simulink model "LQR"  (R2024b)
settings: Solver=VariableStepAuto  StartTime=0.0  StopTime=20  RelTol=1e-3
settings Model: Creator=12625  LastModifiedBy=12625

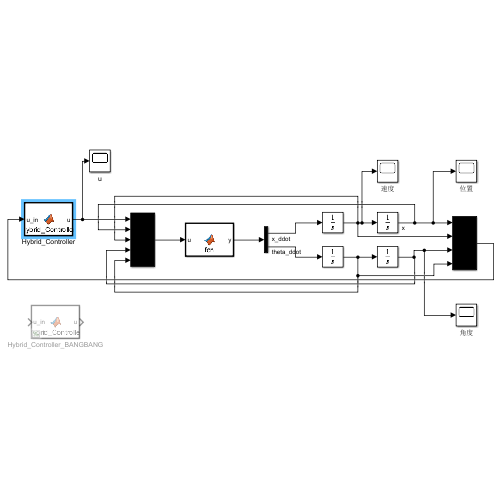
[thumbnail: Simulink's stored preview of the top-level diagram]
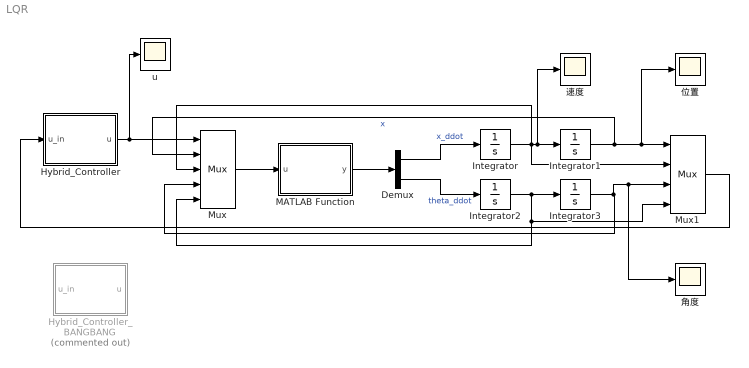
== system LQR ==
  Demux : Demux  Outputs=2
  Hybrid_Controller : MATLAB Function  TreatAsAtomicUnit=on
  Hybrid_Controller_BANGBANG : MATLAB Function  Commented=on  TreatAsAtomicUnit=on
  Integrator : Integrator
  Integrator1 : Integrator
  Integrator2 : Integrator
  Integrator3 : Integrator  InitialCondition=-3.14
  MATLAB Function : MATLAB Function  TreatAsAtomicUnit=on
  Mux : Mux  Inputs=5
  Mux1 : Mux
  u : Scope
  位置 : Scope
  角度 : Scope
  速度 : Scope
  wires:
  Demux/1 -> Integrator/1  "x_ddot"
  Integrator/1 -> Mux1/2, Mux/3, 速度/1, Integrator1/1
  Demux/2 -> Integrator2/1  "theta_ddot"
  Integrator2/1 -> Mux1/4, Mux/5, Integrator3/1
  MATLAB Function/1(y) -> Demux/1
  Integrator1/1 -> 位置/1, Mux1/1, Mux/2  "x"
  Integrator3/1 -> 角度/1, Mux1/3, Mux/4
  Mux1/1 -> Hybrid_Controller/1(u_in)
  Hybrid_Controller/1(u) -> u/1, Mux/1
  Mux/1 -> MATLAB Function/1(u)

== matlab function LQR/MATLAB Function ==
  data: y output; u input
function y = fcn(u)
% 输入 u 包含: [F, x, x_dot, theta, theta_dot]
% 输出 y 包含: [x_ddot, theta_ddot]

% 1. 解包输入
F = u(1);
% x = u(2); % 其实方程里没用到x，只需要速度和角度
x_dot = u(3);
theta = u(4);
theta_dot = u(5);

% 2. 定义参数 (一定要和你的推导一致)
M = 0.5;  % 小车质量
m = 0.2;  % 摆杆质量
l = 0.5;  % 杆长的一半
g = 9.8;
I = 0.005; % 假设均匀杆 I = 1/12*m*(2l)^2 approx

% 3. 写入刚才推导出的公式 (这里用标准形式)
% 这里的公式是为了解出 x_ddot 和 theta_ddot
% 我们可以构建一个矩阵方程 Ax=b 来解，或者直接写解析解
% 为了简单，这里直接写解好的形式 (分母项)

sin_t = sin(theta);
cos_t = cos(theta);
denom = (M+m)*(I+m*l^2) - (m*l*cos_t)^2;

% 分子项
term1 = (I+m*l^2)*F + (I+m*l^2)*m*l*theta_dot^2*sin_t - m*l*cos_t*m*g*sin_t;
term2 = (M+m)*m*g*sin_t - m*l*cos_t*F - m*l*cos_t*m*l*theta_dot^2*sin_t;

x_ddot = term1 / denom;
theta_ddot = term2 / denom;

y = [x_ddot; theta_ddot];

== matlab function LQR/Hybrid_Controller_BANGBANG ==
  data: u output; u_in input
function u = Hybrid_Controller(u_in)
    % 解包输入
    x = u_in(1);
    x_dot = u_in(2);
    theta = u_in(3);     % 原始角度
    theta_dot = u_in(4);
    
    % --- 1. 参数定义 ---
    M = 1.0; m = 0.1; l = 0.5; g = 9.8;
    I_cm = 0.005;
    J = I_cm + m*l^2;
    
    % --- 2. 角度归一化 ---
    theta_norm = mod(theta + pi, 2*pi) - pi;
    
    % --- 3. 能量计算 ---
    E_ref = m * g * l; 
    E_now = 0.5 * J * theta_dot^2 + m * g * l * cos(theta_norm);
    E_err = E_now - E_ref;


    
    % --- 4. 状态机切换逻辑 ---
    if abs(theta_norm) < 0.45
        % === 状态 A: LQR 稳态控制 ===
        K = [-1.0000   ,-3.4655  ,-73.5731  ,-11.5865]; 
        
        state_vec = [x; x_dot; theta_norm; theta_dot];
        u = -K * state_vec;
        
        % LQR 限幅
        u = max(min(u, 20), -20);
        
    else
        % === 状态 B: Swing-Up "慢速安全起摆" ===
        
        % 1. 安全区设置 (保持严格)
        % 只要跑出 0.3米，就开始报警准备救车
        safe_zone_limit = 0.3; 
        
        % 2. 降低推力 (解决 2.5米 的核心)
        % 从 12.0 降到 6.0。
        % 宁可让它多摆 5 秒钟，也不要让车跑太快。
        pump_force = 6.0; 
        
        % 计算推力方向 (Bang-Bang 控制)
        u_swing_direction = -sign(theta_dot * cos(theta_norm));
        u_swing = pump_force * u_swing_direction;
        
        % --- 3. 核心调度 ---
        if abs(x) > safe_zone_limit
            % [红区]：急刹车 (救车模式)
            k_safe_pos = 8.0;  % 强拉力
            k_safe_vel = 5.0;  % 强阻尼
            
            u = - (k_safe_pos * x + k_safe_vel * x_dot);
            
        else
            % [绿区]：带阻尼的起摆 (关键修改!)
            
            % 以前是 u = u_swing; (无阻力)
            % 现在减去速度项 (2.0 * x_dot)。
            % 这就像车轮带点刹车，防止在起摆过程中车速飙升。
            u = u_swing - (2.5 * x_dot); 
        end
        
        % 4. 限幅
        u = max(min(u, 25), -25); 
    end
end

== matlab function LQR/Hybrid_Controller ==
  data: u output; u_in input
function u = Hybrid_Controller(u_in)
    % 解包输入
    x = u_in(1);
    x_dot = u_in(2);
    theta = u_in(3);     
    theta_dot = u_in(4);
    
    % --- 1. 参数定义 (必须与脚本里的黄金参数一致！) ---
    M = 0.5;  % 小车变轻
    m = 0.2;  % 摆杆变重
    l = 0.5;  
    g = 9.8;
    I_cm = 0.005; 
    
    % --- 2. 角度归一化 ---
    theta_norm = mod(theta + pi, 2*pi) - pi;
    
    % --- 3. 能量计算 ---
    J = I_cm + m*l^2;
    E_ref = 0.97*m * g * l; 
    E_now = 0.5 * J * theta_dot^2 + m * g * l * cos(theta_norm);
    
    % --- 4. 状态机切换 ---
    % 只要进入 20度 (0.35 rad) 范围内，就切 LQR
    if abs(theta_norm) < 0.45
        % === 状态 A: LQR 稳态控制 ===
        % 【注意】这里必须用你刚才脚本算出来的新 K 值！
        % 我这里放一个大概的估计值，请用脚本算出的覆盖它
        % 假设 K_new 类似这样 (请务必更新):
        K = [-99.999999999998950,-51.470097958987274,-2.194250822195372e+02,-39.883194125206046]; % <--- 记得替换成 disp(K) 的结果
        
        state_vec = [x; x_dot; theta_norm; theta_dot];
        u = -K * state_vec;
        
        % LQR 阶段也加限幅
        u = max(min(u, 30), -30);
        
    else
        % === 状态 B: Swing-Up "数学软墙 - 温火慢炖版" ===
        
        % --- 1. 能量摆控制 (高效率，低增益) ---
        raw_err = E_now - E_ref;
        
        % [数学技巧1] 误差饱和
        % 使用 atan 将巨大的能量误差平滑地限制在 ±1.5 左右
        % 这保证了无论误差多大，我们请求的力是恒定的，不会暴冲
        E_term = atan(5.0 * raw_err);
        
        % [数学技巧2] 驱动项整形
        % 保持你的要求，用数学公式，不用 bang-bang
        % 使用保号开根号 (Signed Sqrt) 提升低速时的效率
        % 这让它在"慢炖"时也能有效注入能量
        drive_raw = theta_dot * cos(theta_norm);
        drive_term = (drive_raw / (sqrt(abs(drive_raw)) + 0.01)); % 数学上等价于 sign * sqrt
        
        % [关键调整] 降低起摆增益！
        % 之前给 50-60 太大了，导致车必须跑很远。
        % M=0.5 很轻，给 15.0 足够了。让它多摆几圈。
        k_swing = 15.0; 
        
        u_swing = k_swing * E_term * drive_term;
        
        % --- 2. 位置控制 (软控制) ---
        % M=0.5, 我们不再用 40 那种石头硬度，回到柔性控制
        % 让小车像在水里一样，有阻尼，但不是墙
        k_pos = 5.0;  
        k_vel = 3.0;  % 较高的阻尼，吸收震荡
        
        u_pos_linear = - (k_pos * x + k_vel * x_dot);
        
        % --- 3. [核心数学] 高阶多项式软墙 (The Soft Wall) ---
        % 这是实现"短滑轨"的纯数学奥义。
        % 我们构造一个力场：F = -k * (x / limit)^9
        % 当 x = 0.5 时，力极小 (中间自由)。
        % 当 x = 0.8 时，力暴增 (边缘撞墙)。
        % 奇数次幂 (9次方) 自动保留符号，无需 sign 或 if。
        
        x_limit_soft = 0.8; % 你希望的软边界
        k_wall_stiffness = 50.0; % 墙的硬度
        
        % 这是一个纯连续函数
        u_soft_wall = -k_wall_stiffness * (x / x_limit_soft)^9;
        
        % --- 4. 摩擦补偿 ---
        % 使用 atan 代替 sign 实现平滑补偿 (纯数学)
        u_fric = 0.5 * atan(10 * x_dot);
        
        % --- 5. 总输出 ---
        % 起摆力 + 线性回归力 + 软墙力 + 摩擦补偿
        u = u_swing + u_pos_linear + u_soft_wall + u_fric;
        
        % 6. 物理限幅
        u = max(min(u, 30), -30);
    end
end
